simulink model "plant_controller"  (R2014b)
settings: Solver=ode3  StartTime=0.0  StopTime=30  FixedStep=0.001  RelTol=1e-3
values from neighbouring files (symbols this model uses):
  alpha0 = 1.5568e-6    (= 1.5568e-06)    [InitPar.m]
  alpha1 = 6.1744e-6    (= 6.1744e-06)    [InitPar.m]
  beta0 = Pf/we_idle    (= 16.6666666667)    [InitPar.m]
  eta0 = 0.3676    [InitPar.m]    (also in modelerror2.m = par(1))
  eta1 = -1.3443e-4    (= -0.00013443)    [InitPar.m]    (also in modelerror2.m = par(2))
  eta_gen = 0.7    [InitPar.m]
  gamma0 = 0.5313    [InitPar.m]
  gamma1 = 0.0029    [InitPar.m]
  Hl = 42.5e6    (= 42500000)    [InitPar.m]
  I_gen = 15    [InitPar.m]
  inertia_e = 0.23    [InitPar.m]
  kappa = 1.35    [InitPar.m]
  lambda = 1    [InitPar.m]
  LLDR_Ad = sys_d.A    [IdleSpeedControl.m]    (also in controller.mat = [0.598191024839 0.409907216459 0.0269438841076 0.00011532512)
  LLDR_Bd = sys_d.B    [IdleSpeedControl.m]    (also in controller.mat = [-0.0612724695609 0.148424147031 0.16072169034 -0.1539741598)
  LLDR_Cd = sys_d.C    [IdleSpeedControl.m]    (also in controller.mat = [-3.72484254358 -3.027351801 -4.73052845584 -7.08396590617 -)
  LLDR_Dd = sys_d.D    [IdleSpeedControl.m]    (also in controller.mat = 1.97452036747)
  LLDR_Tu = Tu    (= 2.5)    [IdleSpeedControl.m]    (also in controller.mat)
  LLDR_Ty = Ty    (= 127)    [IdleSpeedControl.m]    (also in controller.mat)
  LLDR_u_alphanom = u_alpha_ref    (= 2.5)    [IdleSpeedControl.m]    (also in controller.mat)
  omega_e_ref = 127    [IdleSpeedControl.m]
  p_a = 1e5    (= 100000)    [InitPar.m]
  p_e = 1.05e5    (= 105000)    [InitPar.m]
  p_m_ref = 2.11e4    (= 21100)    [IdleSpeedControl.m]
  R = 0.01    [IdleSpeedControl.m]    (also in InitPar.m = 287)
  sigma0 = 14.67    [InitPar.m]
  T_a = 290    [InitPar.m]
  T_m = 320    [InitPar.m]
  tau_inj_ref = 0.072751    [InitPar.m]
  U_bat = 14    [InitPar.m]
  Vc = 2.48e-4    (= 0.000248)    [InitPar.m]
  Vd = 2.48e-3    (= 0.00248)    [InitPar.m]
  Vm = 0.0057    [InitPar.m]    (also in modelerror.m = par; modelerror2.m = par(3); pm_error.m = simulation_parameters)
  we_idle = 90    [InitPar.m]
  we_tau_inj_ref = we_idle    (= 90)    [InitPar.m]
undefined symbols (not defined in the file or in its folder): meas, sigbuilder_block
settings Model: BufferReuse=off  Creator=kohm  LastModifiedBy=kohm
settings DataIOCC: ExternalInput=[0 2 5.45e-05]  InitialState=[]  SaveFinalState=on  SaveCompleteFinalSimState=on  SaveFormat=StructureWithTime
settings OptimizationCC: InlineParams=on  BufferReuse=off
settings DebuggingCC: InitInArrayFormatMsg=none

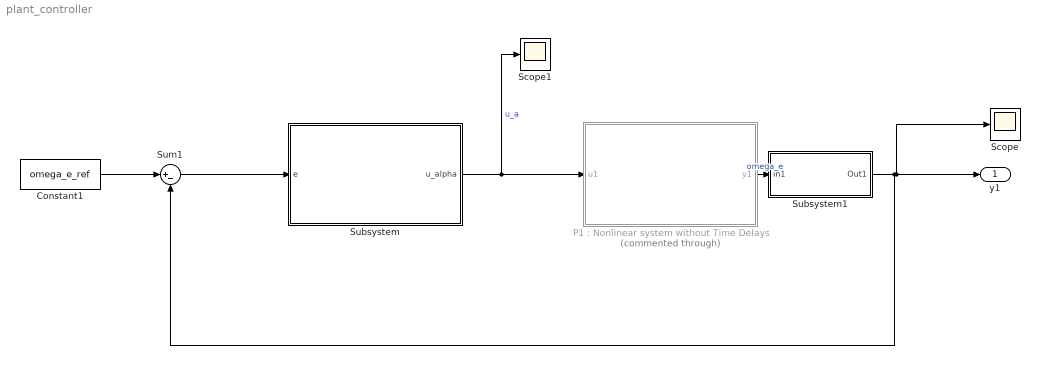
== system plant_controller ==
  Constant1 : Constant  Value=omega_e_ref
  "P1 : Nonlinear system without Time Delays" : Subsystem  Commented=through
  Scope : Scope
      settings: TimeRange=30  YMin=118  YMax=134
  Scope1 : Scope
      settings: TimeRange=4.999000000000002  YMin=1.969  YMax=1.979  SaveName=ScopeData4
  Subsystem : Subsystem
  Subsystem1 : Subsystem
  Sum1 : Sum  Inputs=|+-
  y1 : Outport
  wires:
  "P1 : Nonlinear system without Time Delays"/1(y1) -> Subsystem1/1(In1)  "omega_e"
  Constant1/1 -> Sum1/1
  Subsystem/1(u_alpha) -> Scope1/1, "P1 : Nonlinear system without Time Delays"/1(u1)  "u_a"
  Sum1/1 -> Subsystem/1(e)
  Subsystem1/1(Out1) -> Sum1/2, y1/1, Scope/1

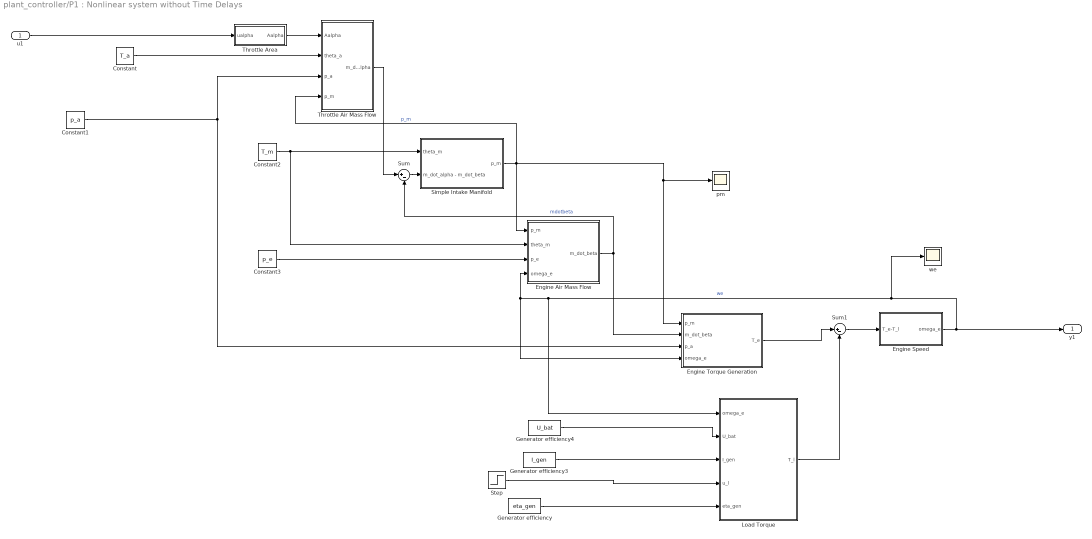
== system plant_controller/P1 : Nonlinear system without Time Delays ==
  u1 : Inport
  Constant : Constant  Value=T_a
  Constant1 : Constant  Value=p_a
  Constant2 : Constant  Value=T_m
  Constant3 : Constant  Value=p_e
  Engine Air Mass Flow : Subsystem
  Engine Speed : Subsystem
  Engine Torque Generation : Subsystem
  Generator efficiency : Constant  Value=eta_gen
  Generator efficiency3 : Constant  Value=I_gen
  Generator efficiency4 : Constant  Value=U_bat
  Load Torque : Subsystem
  "Simple Intake Manifold " : Subsystem
  Step : Step  Time=10  SampleTime=0
  Sum : Sum  Inputs=|+-
  Sum1 : Sum  Inputs=|+-
  Throttle Air Mass Flow : Subsystem
  Throttle Area : Subsystem
  pm : Scope
  "we " : Scope
      settings: SaveName=ScopeData2
  y1 : Outport
  wires:
  u1/1 -> Throttle Area/1(ualpha)
  Throttle Area/1(Aalpha) -> Throttle Air Mass Flow/1(Aalpha)
  Engine Air Mass Flow/1(m_dot_beta) -> Sum/2, Engine Torque Generation/2(m_dot_beta)  "mdotbeta"
  Sum/1 -> "Simple Intake Manifold "/2(m_dot_alpha - m_dot_beta)
  "Simple Intake Manifold "/1("p_m ") -> Engine Air Mass Flow/1(p_m), pm/1, Engine Torque Generation/1(p_m), Throttle Air Mass Flow/4(p_m)  "p_m"
  Engine Torque Generation/1(T_e) -> Sum1/1
  Engine Speed/1(omega_e) -> y1/1, "we "/1, Load Torque/1(omega_e), Engine Air Mass Flow/4(omega_e), Engine Torque Generation/4(omega_e)  "we"
  Constant2/1 -> Engine Air Mass Flow/2(theta_m), "Simple Intake Manifold "/1(theta_m)
  Constant3/1 -> Engine Air Mass Flow/3(p_e)
  Constant/1 -> Throttle Air Mass Flow/2(theta_a)
  Constant1/1 -> Throttle Air Mass Flow/3(p_a), Engine Torque Generation/3(p_a)
  Throttle Air Mass Flow/1(m_dot_alpha) -> Sum/1
  Sum1/1 -> Engine Speed/1("T_e-T_l ")
  Load Torque/1(T_l) -> Sum1/2
  Step/1 -> Load Torque/4(u_l)
  Generator efficiency/1 -> Load Torque/5(eta_gen)
  Generator efficiency4/1 -> Load Torque/2(U_bat)
  Generator efficiency3/1 -> Load Torque/3(I_gen)

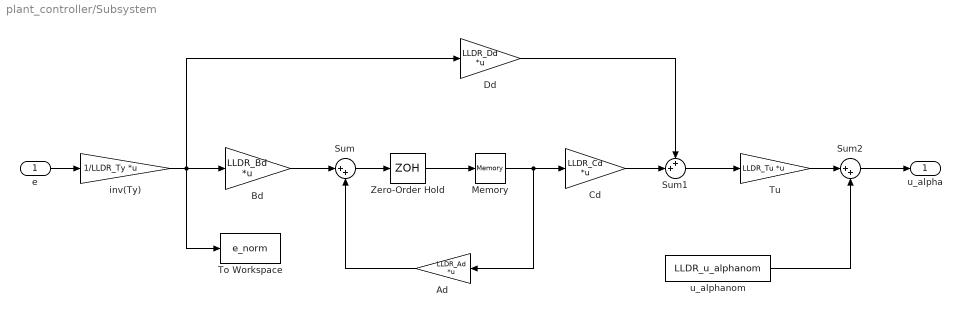
== system plant_controller/Subsystem ==
  e : Inport
  Ad : Gain  Gain=LLDR_Ad  Multiplication=Matrix(K*u)
  Bd : Gain  Gain=LLDR_Bd  Multiplication=Matrix(K*u)
  Cd : Gain  Gain=LLDR_Cd  Multiplication=Matrix(K*u)
  Dd : Gain  Gain=LLDR_Dd  Multiplication=Matrix(K*u)
  Memory : Memory  InheritSampleTime=on
  Sum : Sum  Inputs=|++
  Sum1 : Sum  Inputs=++|
  Sum2 : Sum  Inputs=|++
  To Workspace : ToWorkspace  VariableName=e_norm  SaveFormat=Timeseries  SampleTime=-1
  Tu : Gain  Gain=LLDR_Tu  Multiplication=Matrix(K*u)
  Zero-Order Hold : ZeroOrderHold  SampleTime=0.001
  inv(Ty) : Gain  Gain=1/LLDR_Ty  Multiplication=Matrix(K*u)
  u_alphanom : Constant  Value=LLDR_u_alphanom
  u_alpha : Outport
  wires:
  e/1 -> inv(Ty)/1
  Memory/1 -> Cd/1, Ad/1
  Zero-Order Hold/1 -> Memory/1
  Sum/1 -> Zero-Order Hold/1
  Cd/1 -> Sum1/2
  Dd/1 -> Sum1/1
  inv(Ty)/1 -> Bd/1, Dd/1, To Workspace/1
  Bd/1 -> Sum/1
  Sum1/1 -> Tu/1
  Tu/1 -> Sum2/1
  u_alphanom/1 -> Sum2/2
  Sum2/1 -> u_alpha/1
  Ad/1 -> Sum/2

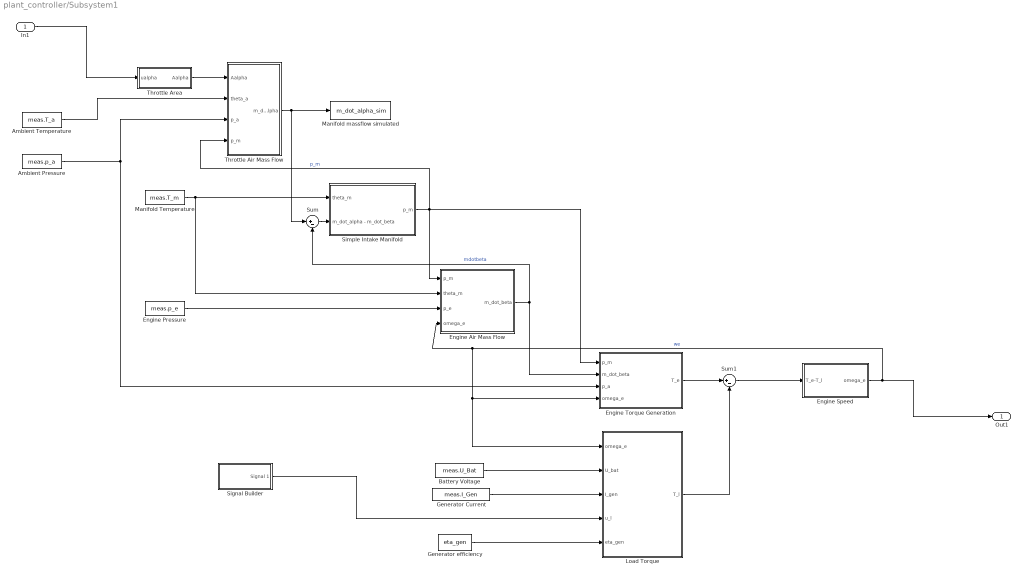
== system plant_controller/Subsystem1 ==
  In1 : Inport
  Ambient Pressure : FromWorkspace  VariableName=meas.p_a  SampleTime=0
  Ambient Temperature : FromWorkspace  VariableName=meas.T_a  SampleTime=0
  Battery Voltage : FromWorkspace  VariableName=meas.U_Bat  SampleTime=0
  Engine Air Mass Flow : Subsystem
  Engine Pressure : FromWorkspace  VariableName=meas.p_e  SampleTime=0
  Engine Speed : Subsystem
  Engine Torque Generation : Subsystem
  Generator Current : FromWorkspace  VariableName=meas.I_Gen  SampleTime=0
  Generator efficiency : Constant  Value=eta_gen
  Load Torque : Subsystem
  Manifold Temperature : FromWorkspace  VariableName=meas.T_m  SampleTime=0
  Manifold massflow simulated : ToWorkspace  VariableName=m_dot_alpha_sim  SaveFormat=Timeseries  SampleTime=-1
  Signal Builder : Subsystem  Tag=STV Subsys  LoadFcn=sigbuilder_block('load',[437.6 199.2 550.4 400 ]);  StartFcn=sigbuilder_block('start');  StopFcn=sigbuilder_block('stop');  ClipboardFcn=sigbuilder_block('clipboard');  mask(Sigbuilder block){}
      mask help: Simulink:masks:SigbuilderBlock_MD
      mask init:
      | if ~strcmp(get_param(bdroot(gcbh),'SimulationStatus'),'stopped') tuvar = sigbuilder_block('maskInit'); end
      settings: CopyFcn=sigbuilder_block('copy');  DeleteFcn=sigbuilder_block('delete');  ModelCloseFcn=sigbuilder_block('modelClose');  PreSaveFcn=sigbuilder_block('preSave');  PauseFcn=sigbuilder_block('pause');  ContinueFcn=sigbuilder_block('continue');  NameChangeFcn=sigbuilder_block('namechange');  OpenFcn=sigbuilder_block('open',[437.6 199.2 550.4 400 ]);  CloseFcn=sigbuilder_block('close');
      mask Display: plot(0, 0, 100, 100,[2, 2, 32, 32, 2], [68, 8, 8, 68, 68],[32, 2], [38, 38], [32, 19, 2],[53, 60, 44], [32, 17, 17, 2],[16, 16, 31, 31]);txt = getActiveGroup(gcbh);text(2, 100, txt,'verticalAlignment', 'top');
  "Simple Intake Manifold " : Subsystem
  Sum : Sum  Inputs=|+-
  Sum1 : Sum  Inputs=|+-
  Throttle Air Mass Flow : Subsystem
  Throttle Area : Subsystem
  Out1 : Outport
  wires:
  Throttle Area/1(Aalpha) -> Throttle Air Mass Flow/1(Aalpha)
  Engine Air Mass Flow/1(m_dot_beta) -> Sum/2, Engine Torque Generation/2(m_dot_beta)  "mdotbeta"
  Sum/1 -> "Simple Intake Manifold "/2(m_dot_alpha - m_dot_beta)
  "Simple Intake Manifold "/1("p_m ") -> Engine Air Mass Flow/1(p_m), Engine Torque Generation/1(p_m), Throttle Air Mass Flow/4(p_m)  "p_m"
  Engine Torque Generation/1(T_e) -> Sum1/1
  Load Torque/1(T_l) -> Sum1/2
  Sum1/1 -> Engine Speed/1("T_e-T_l ")
  Engine Speed/1(omega_e) -> Out1/1, Engine Air Mass Flow/4(omega_e), Engine Torque Generation/4(omega_e), Load Torque/1(omega_e)  "we"
  Signal Builder/1(Signal 1) -> Load Torque/4(u_l)
  In1/1 -> Throttle Area/1(ualpha)
  Manifold Temperature/1 -> Engine Air Mass Flow/2(theta_m), "Simple Intake Manifold "/1(theta_m)
  Battery Voltage/1 -> Load Torque/2(U_bat)
  Generator Current/1 -> Load Torque/3(I_gen)
  Engine Pressure/1 -> Engine Air Mass Flow/3(p_e)
  Ambient Temperature/1 -> Throttle Air Mass Flow/2(theta_a)
  Ambient Pressure/1 -> Engine Torque Generation/3(p_a), Throttle Air Mass Flow/3(p_a)
  Generator efficiency/1 -> Load Torque/5(eta_gen)
  Throttle Air Mass Flow/1(m_dot_alpha) -> Sum/1, Manifold massflow simulated/1

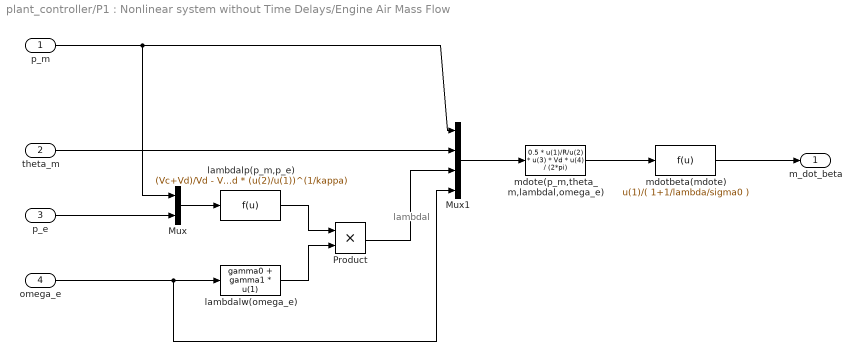
== system plant_controller/P1 : Nonlinear system without Time Delays/Engine Air Mass Flow ==
  note: lambdal
  p_m : Inport
  theta_m : Inport  Port=2
  p_e : Inport  Port=3
  omega_e : Inport  Port=4
  Mux : Mux  Inputs=2
  Mux1 : Mux
  Product : Product
  lambdalp(p_m,p_e) : Fcn  Expr=(Vc+Vd)/Vd - Vc/Vd * (u(2)/u(1))^(1/kappa)
  lambdalw(omega_e) : Fcn  Expr=gamma0 + gamma1 * u(1)
  mdotbeta(mdote) : Fcn  Expr=u(1)/( 1+1/lambda/sigma0 )
  mdote(p_m,theta_m,lambdal,omega_e) : Fcn  Expr=0.5 * u(1)/R/u(2) * u(3) * Vd * u(4) / (2*pi)
  m_dot_beta : Outport
  wires:
  lambdalw(omega_e)/1 -> Product/2
  lambdalp(p_m,p_e)/1 -> Product/1
  Product/1 -> Mux1/3
  Mux/1 -> lambdalp(p_m,p_e)/1
  p_e/1 -> Mux/2
  p_m/1 -> Mux/1, Mux1/1
  omega_e/1 -> Mux1/4, lambdalw(omega_e)/1
  Mux1/1 -> mdote(p_m,theta_m,lambdal,omega_e)/1
  theta_m/1 -> Mux1/2
  mdote(p_m,theta_m,lambdal,omega_e)/1 -> mdotbeta(mdote)/1
  mdotbeta(mdote)/1 -> m_dot_beta/1

== system plant_controller/P1 : Nonlinear system without Time Delays/Engine Speed ==
  "T_e-T_l " : Inport
  dwe/dt : Integrator  InitialCondition=omega_e_ref  LowerSaturationLimit=0  ContinuousStateAttributes='w_e'
  inverse rotational inertia : Gain  Gain=1/inertia_e
  omega_e : Outport
  wires:
  "T_e-T_l "/1 -> inverse rotational inertia/1
  inverse rotational inertia/1 -> dwe/dt/1
  dwe/dt/1 -> omega_e/1

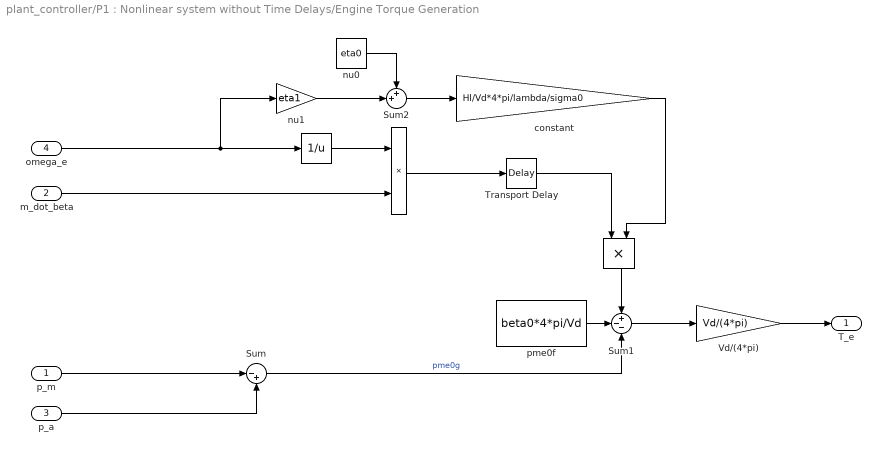
== system plant_controller/P1 : Nonlinear system without Time Delays/Engine Torque Generation ==
  p_m : Inport
  m_dot_beta : Inport  Port=2
  p_a : Inport  Port=3
  omega_e : Inport  Port=4
  " " : Product
  " " : Math  Operator=reciprocal  SaturateOnIntegerOverflow=on
  " " : Product
  Sum : Sum  Inputs=|-+
  Sum1 : Sum  Inputs=+--
  Sum2 : Sum  Inputs=++|
  Transport Delay : TransportDelay  DelayTime=0.06
  Vd/(4*pi) : Gain  Gain=Vd/(4*pi)
  constant : Gain  Gain=Hl/Vd*4*pi/lambda/sigma0
  "nu0 " : Constant  Value=eta0
  "nu1 " : Gain  Gain=eta1
  pme0f : Constant  Value=beta0*4*pi/Vd
  T_e : Outport
  wires:
  Vd/(4*pi)/1 -> T_e/1
  p_m/1 -> Sum/1
  Sum1/1 -> Vd/(4*pi)/1
  Sum/1 -> Sum1/3  "pme0g"
  pme0f/1 -> Sum1/2
  "nu0 "/1 -> Sum2/1
  "nu1 "/1 -> Sum2/2
  Sum2/1 -> constant/1
  constant/1 -> " "/2
  " "/1 -> Sum1/1
  " "/1 -> " "/1
  m_dot_beta/1 -> " "/2
  " "/1 -> Transport Delay/1
  p_a/1 -> Sum/2
  omega_e/1 -> " "/1, "nu1 "/1
  Transport Delay/1 -> " "/1

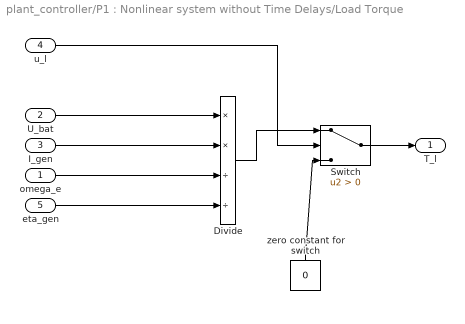
== system plant_controller/P1 : Nonlinear system without Time Delays/Load Torque ==
  omega_e : Inport
  U_bat : Inport  Port=2
  I_gen : Inport  Port=3
  u_l : Inport  Port=4
  eta_gen : Inport  Port=5
  " zero constant for switch" : Constant  Value=0
  Divide : Product  Inputs=**//
  Switch : Switch  Criteria=u2 > Threshold
  T_l : Outport
  wires:
  U_bat/1 -> Divide/1
  I_gen/1 -> Divide/2
  omega_e/1 -> Divide/3
  eta_gen/1 -> Divide/4
  Divide/1 -> Switch/1
  u_l/1 -> Switch/2
  Switch/1 -> T_l/1
  " zero constant for switch"/1 -> Switch/3

== system plant_controller/P1 : Nonlinear system without Time Delays/Simple Intake Manifold  ==
  theta_m : Inport
  m_dot_alpha - m_dot_beta : Inport  Port=2
  Product : Product  Inputs=3
  R/Vm : Constant  Value=R/Vm
  p_m_integrator : Integrator  InitialCondition=p_m_ref  ContinuousStateAttributes='p_m'
  "p_m " : Outport
  wires:
  p_m_integrator/1 -> "p_m "/1  "p_m"
  Product/1 -> p_m_integrator/1
  theta_m/1 -> Product/3
  m_dot_alpha - m_dot_beta/1 -> Product/2
  R/Vm/1 -> Product/1

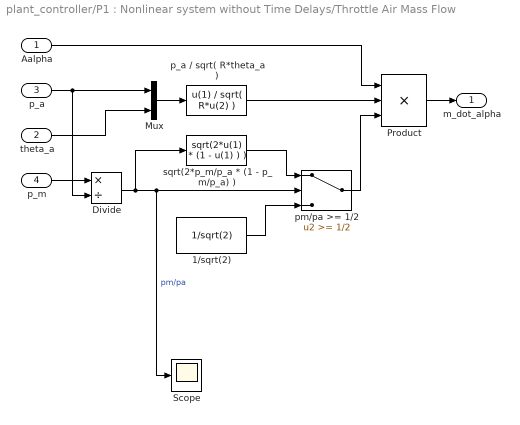
== system plant_controller/P1 : Nonlinear system without Time Delays/Throttle Air Mass Flow ==
  Aalpha : Inport
  theta_a : Inport  Port=2
  p_a : Inport  Port=3
  p_m : Inport  Port=4
  1/sqrt(2) : Constant  Value=1/sqrt(2)
  Divide : Product  Inputs=*/
  Mux : Mux  Inputs=2
  Product : Product  Inputs=3
  Scope : Scope
      settings: SaveName=ScopeData3
  p_a / sqrt( R*theta_a ) : Fcn  Expr=u(1) / sqrt( R*u(2) )
  pm/pa >= 1/2 : Switch  Threshold=1/2
  sqrt(2*p_m/p_a * (1 - p_m/p_a) ) : Fcn  Expr=sqrt(2*u(1) * (1 - u(1) ) )
  m_dot_alpha : Outport
  wires:
  Mux/1 -> p_a / sqrt( R*theta_a )/1
  theta_a/1 -> Mux/2
  p_a / sqrt( R*theta_a )/1 -> Product/2
  p_a/1 -> Mux/1, Divide/2
  p_m/1 -> Divide/1
  Divide/1 -> Scope/1, pm/pa >= 1/2/2, sqrt(2*p_m/p_a * (1 - p_m/p_a) )/1  "pm/pa"
  1/sqrt(2)/1 -> pm/pa >= 1/2/3
  pm/pa >= 1/2/1 -> Product/3
  sqrt(2*p_m/p_a * (1 - p_m/p_a) )/1 -> pm/pa >= 1/2/1
  Product/1 -> m_dot_alpha/1
  Aalpha/1 -> Product/1

== system plant_controller/P1 : Nonlinear system without Time Delays/Throttle Area ==
  ualpha : Inport
  Aalpha(ualpha) : Fcn  Expr=alpha0 + alpha1 * u(1)
  Aalpha : Outport
  wires:
  ualpha/1 -> Aalpha(ualpha)/1
  Aalpha(ualpha)/1 -> Aalpha/1

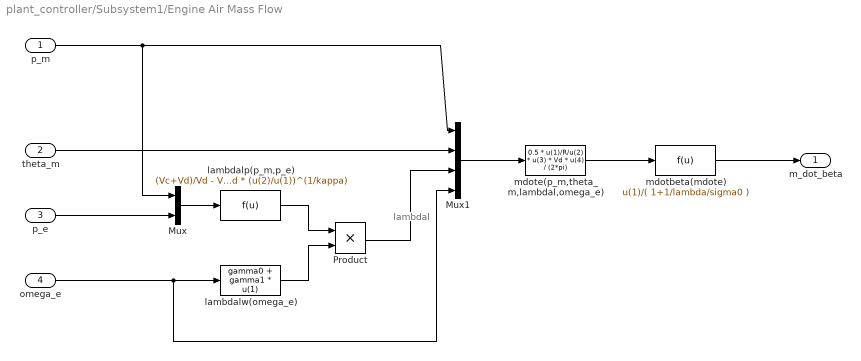
== system plant_controller/Subsystem1/Engine Air Mass Flow ==
  note: lambdal
  p_m : Inport
  theta_m : Inport  Port=2
  p_e : Inport  Port=3
  omega_e : Inport  Port=4
  Mux : Mux  Inputs=2
  Mux1 : Mux
  Product : Product
  lambdalp(p_m,p_e) : Fcn  Expr=(Vc+Vd)/Vd - Vc/Vd * (u(2)/u(1))^(1/kappa)
  lambdalw(omega_e) : Fcn  Expr=gamma0 + gamma1 * u(1)
  mdotbeta(mdote) : Fcn  Expr=u(1)/( 1+1/lambda/sigma0 )
  mdote(p_m,theta_m,lambdal,omega_e) : Fcn  Expr=0.5 * u(1)/R/u(2) * u(3) * Vd * u(4) / (2*pi)
  m_dot_beta : Outport
  wires:
  lambdalw(omega_e)/1 -> Product/2
  lambdalp(p_m,p_e)/1 -> Product/1
  Product/1 -> Mux1/3
  Mux/1 -> lambdalp(p_m,p_e)/1
  p_e/1 -> Mux/2
  p_m/1 -> Mux/1, Mux1/1
  omega_e/1 -> Mux1/4, lambdalw(omega_e)/1
  Mux1/1 -> mdote(p_m,theta_m,lambdal,omega_e)/1
  theta_m/1 -> Mux1/2
  mdote(p_m,theta_m,lambdal,omega_e)/1 -> mdotbeta(mdote)/1
  mdotbeta(mdote)/1 -> m_dot_beta/1

== system plant_controller/Subsystem1/Engine Speed ==
  "T_e-T_l " : Inport
  dwe/dt : Integrator  InitialCondition=meas.omega_e.signals.values(1)  LowerSaturationLimit=0  ContinuousStateAttributes='w_e'
  inverse rotational inertia : Gain  Gain=1/inertia_e
  omega_e : Outport
  wires:
  "T_e-T_l "/1 -> inverse rotational inertia/1
  inverse rotational inertia/1 -> dwe/dt/1
  dwe/dt/1 -> omega_e/1

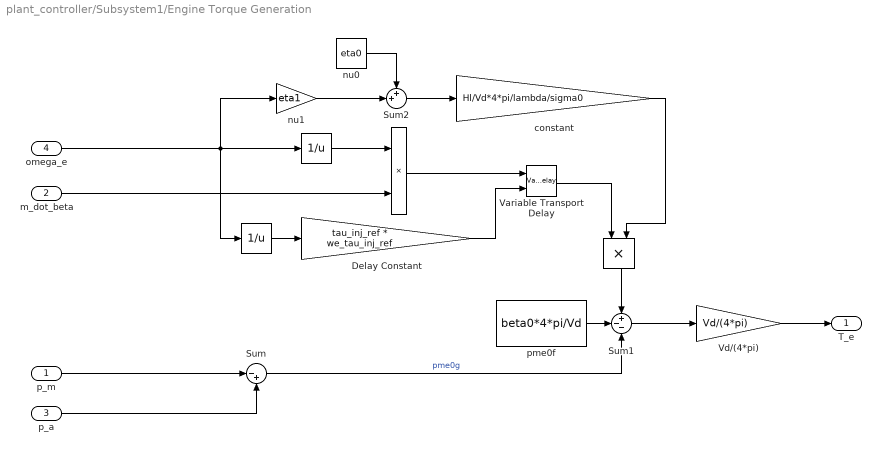
== system plant_controller/Subsystem1/Engine Torque Generation ==
  p_m : Inport
  m_dot_beta : Inport  Port=2
  p_a : Inport  Port=3
  omega_e : Inport  Port=4
  " " : Math  Operator=reciprocal  SaturateOnIntegerOverflow=on
  " " : Product
  " " : Math  Operator=reciprocal  SaturateOnIntegerOverflow=on
  " " : Product
  Delay Constant : Gain  Gain=tau_inj_ref * we_tau_inj_ref
  Sum : Sum  Inputs=|-+
  Sum1 : Sum  Inputs=+--
  Sum2 : Sum  Inputs=++|
  Variable Transport Delay : VariableTransportDelay  MaximumDelay=10  InitialOutput=1/we_idle*0.002  MaximumPoints=10240
  Vd/(4*pi) : Gain  Gain=Vd/(4*pi)
  constant : Gain  Gain=Hl/Vd*4*pi/lambda/sigma0
  "nu0 " : Constant  Value=eta0
  "nu1 " : Gain  Gain=eta1
  pme0f : Constant  Value=beta0*4*pi/Vd
  T_e : Outport
  wires:
  Vd/(4*pi)/1 -> T_e/1
  p_m/1 -> Sum/1
  Sum1/1 -> Vd/(4*pi)/1
  Sum/1 -> Sum1/3  "pme0g"
  pme0f/1 -> Sum1/2
  "nu0 "/1 -> Sum2/1
  "nu1 "/1 -> Sum2/2
  Sum2/1 -> constant/1
  constant/1 -> " "/2
  " "/1 -> Sum1/1
  " "/1 -> " "/1
  Delay Constant/1 -> Variable Transport Delay/2
  m_dot_beta/1 -> " "/2
  " "/1 -> Variable Transport Delay/1
  p_a/1 -> Sum/2
  omega_e/1 -> " "/1, " "/1, "nu1 "/1
  " "/1 -> Delay Constant/1
  Variable Transport Delay/1 -> " "/1

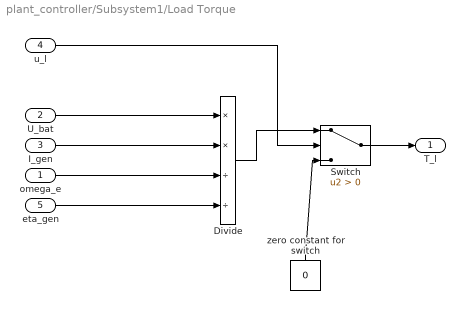
== system plant_controller/Subsystem1/Load Torque ==
  omega_e : Inport
  U_bat : Inport  Port=2
  I_gen : Inport  Port=3
  u_l : Inport  Port=4
  eta_gen : Inport  Port=5
  " zero constant for switch" : Constant  Value=0
  Divide : Product  Inputs=**//
  Switch : Switch  Criteria=u2 > Threshold
  T_l : Outport
  wires:
  U_bat/1 -> Divide/1
  I_gen/1 -> Divide/2
  omega_e/1 -> Divide/3
  eta_gen/1 -> Divide/4
  Divide/1 -> Switch/1
  u_l/1 -> Switch/2
  Switch/1 -> T_l/1
  " zero constant for switch"/1 -> Switch/3

== system plant_controller/Subsystem1/Signal Builder ==
  Demux : Demux  Tag=STV Demux  Outputs=1
  FromWs : FromWorkspace  Tag=STV FromWs  VariableName=tuvar  SampleTime=0
      SigBuilderData=|
      | common.afterFinalStr = 'Extrapolate'
      | common.sampleTime = 0
      | dataSet.timeRange = [0 10]
      | dataSet.name = 'Group 1'
      | sbobj.Groups.Name = 'Group 1'
      | sbobj.Groups.Signals.Name = 'Signal 1'
      | sbobj.Groups.Signals.XData = [0 4 4 6 6 10]
      | sbobj.Groups.Signals.YData = [0 0.45 1 1 0 0]
  Signal 1 : Outport  Tag=STV Outport
  wires:
  Demux/1 -> Signal 1/1
  FromWs/1 -> Demux/1

== system plant_controller/Subsystem1/Simple Intake Manifold  ==
  theta_m : Inport
  m_dot_alpha - m_dot_beta : Inport  Port=2
  Product : Product  Inputs=3
  R/Vm : Constant  Value=R/Vm
  p_m_integrator : Integrator  InitialCondition=meas.p_m.signals.values(1)
  "p_m " : Outport
  wires:
  p_m_integrator/1 -> "p_m "/1  "p_m"
  Product/1 -> p_m_integrator/1
  theta_m/1 -> Product/3
  m_dot_alpha - m_dot_beta/1 -> Product/2
  R/Vm/1 -> Product/1

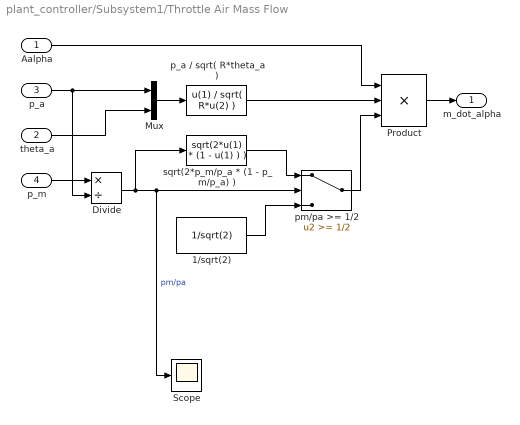
== system plant_controller/Subsystem1/Throttle Air Mass Flow ==
  Aalpha : Inport
  theta_a : Inport  Port=2
  p_a : Inport  Port=3
  p_m : Inport  Port=4
  1/sqrt(2) : Constant  Value=1/sqrt(2)
  Divide : Product  Inputs=*/
  Mux : Mux  Inputs=2
  Product : Product  Inputs=3
  Scope : Scope
      settings: SaveName=ScopeData3
  p_a / sqrt( R*theta_a ) : Fcn  Expr=u(1) / sqrt( R*u(2) )
  pm/pa >= 1/2 : Switch  Threshold=1/2
  sqrt(2*p_m/p_a * (1 - p_m/p_a) ) : Fcn  Expr=sqrt(2*u(1) * (1 - u(1) ) )
  m_dot_alpha : Outport
  wires:
  Mux/1 -> p_a / sqrt( R*theta_a )/1
  theta_a/1 -> Mux/2
  p_a / sqrt( R*theta_a )/1 -> Product/2
  p_a/1 -> Mux/1, Divide/2
  p_m/1 -> Divide/1
  Divide/1 -> Scope/1, pm/pa >= 1/2/2, sqrt(2*p_m/p_a * (1 - p_m/p_a) )/1  "pm/pa"
  1/sqrt(2)/1 -> pm/pa >= 1/2/3
  pm/pa >= 1/2/1 -> Product/3
  sqrt(2*p_m/p_a * (1 - p_m/p_a) )/1 -> pm/pa >= 1/2/1
  Product/1 -> m_dot_alpha/1
  Aalpha/1 -> Product/1

== system plant_controller/Subsystem1/Throttle Area ==
  ualpha : Inport
  Aalpha(ualpha) : Fcn  Expr=alpha0 + alpha1 * u(1)
  Aalpha : Outport
  wires:
  ualpha/1 -> Aalpha(ualpha)/1
  Aalpha(ualpha)/1 -> Aalpha/1
